simulink model "EPT"  (R2019b)
settings: Solver=FixedStepDiscrete  StartTime=0.0  StopTime=5  FixedStep=0.005  RelTol=1e-3  EnableMultiTasking=on
PreLoadFcn:
  | try, model_open; catch, disp('Error occurred while executing model pre-load callback: model_open.m'); disp('Please assure that the MATLAB working directory is set to the model directory before opening.'); end
InitFcn:
  | try, model_open; catch, end
undefined symbols (not defined in the file or in its folder): Bridge, GCM, H, ln, raptor_get_param_eval, raptor_get_safe_string, raptor_xcp_function
libraries: Raptor_lib x2810, simulink x374, hdlsllib x19
(part 28 of 45)

== system EPT/Foreground_TimeBase_5ms/CAN/CAN1_exec/BCU-CMU/CMU_Task/Tx C0-C3 ==
  Trigger : TriggerPort  VariantControl=Variant  PortDimensions=1
  Constant3 : Constant  Value=4
  Constant4 : Constant  Value=hex2dec('A0')
  Constant5 : Constant  Value=hex2dec('C0')
  raptor_can_txmsg : Raptor_lib/CAN/raptor_can_txmsg  canDefinition=struct('dbcFile', 'CMU_CMD.dbc','message', 'HostReadCMD','comment', '','signals', {{'CMU_ID','Offset','Function_Index','ID','LifeCycle'}},'enabled', [ 1 1 1 1 1;],'canBus', '''CAN1''','messageID', [ 16838272;],'idMask', [ 536870911;],'payloadMask', [],'payloadValue', [],'period', [ 0;],'mailbox', '','queueSize', [ 1;],'label', [ 1;],'ver', [ 2;],'showID', [ 0;],'showRaw', [ 0;],'fill', [ 0;],'editID', [ 0;],'signalOrder', [ 2;])  canBus='CAN1'  queueSize=1  payloadMask=[]  payloadValue=[]  period=0  showID=0  label=1  idMask=hex2dec('1FFFFFFF')  fill=0  id=16838272  showRaw=0  signalOrder=2  signalInfo={{struct('Name', 'CMU_ID','Startbit', [ 0;],'SignalSize', [ 8;],'ByteOrder', 'LittleEndian','ValueType', 'UNSIGNED','Class', 'uint8','Signed', [ 0;],'Factor', [ 1;],'Offset', [ 0;],'Min', [ 0;],'Max', [ 0;],'Units', '','Comment', '','StartBit', [ 0;]),struct('Name', 'Offset','Startbit', [ 0;],'SignalSize', [ 8;],'ByteOrder', 'LittleEndian','ValueType', 'UNSIGNED','Class', 'uint8','Signed', [ 0;],'Factor', [ 1;],'Offset', [ 0;],'Min', [ 0;],'Max', [ 0;],'Units', '','Comment', '','StartBit', [ 32;]),struct('Name', 'Function_Index','Startbit', [ 0;],'SignalSize', [ 8;],'ByteOrder', 'LittleEndian','ValueType', 'UNSIGNED','Class', 'uint8','Signed', [ 0;],'Factor', [ 1;],'Offset', [ 0;],'Min', [ 0;],'Max', [ 0;],'Units', '','Comment', '','StartBit', [ 40;]),struct('Name', 'LifeCycle','Startbit', [ 0;],'SignalSize', [ 4;],'ByteOrder', 'LittleEndian','ValueType', 'UNSIGNED','Class', 'uint8','Signed', [ 0;],'Factor', [ 1;],'Offset', [ 0;],'Min', [ 0;],'Max', [ 0;],'Units', '','Comment', '','StartBit', [ 60;]),struct('Name', 'ID','Startbit', [ 0;],'SignalSize', [ 4;],'ByteOrder', 'LittleEndian','ValueType', 'UNSIGNED','Class', 'uint8','Signed', [ 0;],'Factor', [ 1;],'Offset', [ 0;],'Min', [ 0;],'Max', [ 0;],'Units', '','Comment', '','StartBit', [ 56;])}}
      settings: SourceProductName=Raptor
  raptor_data_read2 : Raptor_lib/Data Storage/raptor_data_read  dataName='EPT_RDCMD_RC'  dataShape=Scalar  idxSource=Input  idxRow=1  idxCol=1
      settings: SourceProductName=Raptor
  raptor_data_read4 : Raptor_lib/Data Storage/raptor_data_read  dataName='EPT_RDCMD_HOST_ID'  dataShape=Scalar  idxSource=Input  idxRow=1  idxCol=1
      settings: SourceProductName=Raptor
  wires:
  raptor_data_read4/1 -> raptor_can_txmsg/4  "ID"
  Constant5/1 -> raptor_can_txmsg/3  "Function_Index"
  raptor_data_read2/1 -> raptor_can_txmsg/5  "LifeCycle"
  Constant4/1 -> raptor_can_txmsg/1  "CMU_ID"
  Constant3/1 -> raptor_can_txmsg/2  "Offset"

== system EPT/Foreground_TimeBase_5ms/CAN/CAN1_exec/BCU-CMU/CMU_Task/Tx C4-C7 ==
  Trigger : TriggerPort  VariantControl=Variant  PortDimensions=1
  Constant3 : Constant  Value=4
  Constant4 : Constant  Value=hex2dec('A0')
  Constant5 : Constant  Value=hex2dec('C4')
  raptor_can_txmsg : Raptor_lib/CAN/raptor_can_txmsg  canDefinition=struct('dbcFile', 'CMU_CMD.dbc','message', 'HostReadCMD','comment', '','signals', {{'CMU_ID','Offset','Function_Index','ID','LifeCycle'}},'enabled', [ 1 1 1 1 1;],'canBus', '''CAN1''','messageID', [ 16838272;],'idMask', [ 536870911;],'payloadMask', [],'payloadValue', [],'period', [ 0;],'mailbox', '','queueSize', [ 1;],'label', [ 1;],'ver', [ 2;],'showID', [ 0;],'showRaw', [ 0;],'fill', [ 0;],'editID', [ 0;],'signalOrder', [ 2;])  canBus='CAN1'  queueSize=1  payloadMask=[]  payloadValue=[]  period=0  showID=0  label=1  idMask=hex2dec('1FFFFFFF')  fill=0  id=16838272  showRaw=0  signalOrder=2  signalInfo={{struct('Name', 'CMU_ID','Startbit', [ 0;],'SignalSize', [ 8;],'ByteOrder', 'LittleEndian','ValueType', 'UNSIGNED','Class', 'uint8','Signed', [ 0;],'Factor', [ 1;],'Offset', [ 0;],'Min', [ 0;],'Max', [ 0;],'Units', '','Comment', '','StartBit', [ 0;]),struct('Name', 'Offset','Startbit', [ 0;],'SignalSize', [ 8;],'ByteOrder', 'LittleEndian','ValueType', 'UNSIGNED','Class', 'uint8','Signed', [ 0;],'Factor', [ 1;],'Offset', [ 0;],'Min', [ 0;],'Max', [ 0;],'Units', '','Comment', '','StartBit', [ 32;]),struct('Name', 'Function_Index','Startbit', [ 0;],'SignalSize', [ 8;],'ByteOrder', 'LittleEndian','ValueType', 'UNSIGNED','Class', 'uint8','Signed', [ 0;],'Factor', [ 1;],'Offset', [ 0;],'Min', [ 0;],'Max', [ 0;],'Units', '','Comment', '','StartBit', [ 40;]),struct('Name', 'LifeCycle','Startbit', [ 0;],'SignalSize', [ 4;],'ByteOrder', 'LittleEndian','ValueType', 'UNSIGNED','Class', 'uint8','Signed', [ 0;],'Factor', [ 1;],'Offset', [ 0;],'Min', [ 0;],'Max', [ 0;],'Units', '','Comment', '','StartBit', [ 60;]),struct('Name', 'ID','Startbit', [ 0;],'SignalSize', [ 4;],'ByteOrder', 'LittleEndian','ValueType', 'UNSIGNED','Class', 'uint8','Signed', [ 0;],'Factor', [ 1;],'Offset', [ 0;],'Min', [ 0;],'Max', [ 0;],'Units', '','Comment', '','StartBit', [ 56;])}}
      settings: SourceProductName=Raptor
  raptor_data_read2 : Raptor_lib/Data Storage/raptor_data_read  dataName='EPT_RDCMD_RC'  dataShape=Scalar  idxSource=Input  idxRow=1  idxCol=1
      settings: SourceProductName=Raptor
  raptor_data_read4 : Raptor_lib/Data Storage/raptor_data_read  dataName='EPT_RDCMD_HOST_ID'  dataShape=Scalar  idxSource=Input  idxRow=1  idxCol=1
      settings: SourceProductName=Raptor
  wires:
  raptor_data_read4/1 -> raptor_can_txmsg/4  "ID"
  Constant5/1 -> raptor_can_txmsg/3  "Function_Index"
  raptor_data_read2/1 -> raptor_can_txmsg/5  "LifeCycle"
  Constant4/1 -> raptor_can_txmsg/1  "CMU_ID"
  Constant3/1 -> raptor_can_txmsg/2  "Offset"

== system EPT/Foreground_TimeBase_5ms/CAN/CAN1_exec/IVT/CountTrigger/CycleTrigger ==
  In1 : Inport
  In2 : Inport  Port=2
  Add : Sum
  Add1 : Sum
  Add2 : Sum  Inputs=+-
  Constant1 : Constant
  Constant2 : Constant  Value=0
  Constant3 : Constant
  Data Type Conversion1 : DataTypeConversion
  Data Type Conversion2 : DataTypeConversion
  Display : Display
  Relational Operator1 : RelationalOperator  OutDataTypeStr=boolean  RndMeth=Simplest
  Scope : Scope
  Scope1 : Scope
  Scope2 : Scope
  Switch : Switch  Threshold=1
  Unit Delay : UnitDelay  SampleTime=-1  HasFrameUpgradeWarning=on
  Unit Delay1 : UnitDelay  SampleTime=-1  HasFrameUpgradeWarning=on
  Trigger : Outport  VectorParamsAs1DForOutWhenUnconnected=off
  wires:
  Constant3/1 -> Add2/2
  In2/1 -> Add2/1
  Add2/1 -> Data Type Conversion1/1
  Data Type Conversion2/1 -> Switch/2, Add/2
  Constant2/1 -> Switch/3
  Data Type Conversion1/1 -> Relational Operator1/2
  Relational Operator1/1 -> Trigger/1, Scope2/1
  Constant1/1 -> Add1/2
  Unit Delay1/1 -> Add1/1
  Add1/1 -> Display/1, Unit Delay1/1, Scope/1
  Switch/1 -> Unit Delay/1, Scope1/1, Relational Operator1/1
  Unit Delay/1 -> Add/1
  In1/1 -> Data Type Conversion2/1
  Add/1 -> Switch/1

== system EPT/Foreground_TimeBase_5ms/CAN/CAN1_exec/IVT/CountTrigger1/CycleTrigger ==
  In1 : Inport
  In2 : Inport  Port=2
  Add : Sum
  Add1 : Sum
  Add2 : Sum  Inputs=+-
  Constant1 : Constant
  Constant2 : Constant  Value=0
  Constant3 : Constant
  Data Type Conversion1 : DataTypeConversion
  Data Type Conversion2 : DataTypeConversion
  Display : Display
  Relational Operator1 : RelationalOperator  OutDataTypeStr=boolean  RndMeth=Simplest
  Scope : Scope
  Scope1 : Scope
  Scope2 : Scope
  Switch : Switch  Threshold=1
  Unit Delay : UnitDelay  SampleTime=-1  HasFrameUpgradeWarning=on
  Unit Delay1 : UnitDelay  SampleTime=-1  HasFrameUpgradeWarning=on
  Trigger : Outport  VectorParamsAs1DForOutWhenUnconnected=off
  wires:
  Add/1 -> Switch/1
  In1/1 -> Data Type Conversion2/1
  Unit Delay/1 -> Add/1
  Switch/1 -> Relational Operator1/1, Scope1/1, Unit Delay/1
  Add1/1 -> Scope/1, Unit Delay1/1, Display/1
  Unit Delay1/1 -> Add1/1
  Constant1/1 -> Add1/2
  Relational Operator1/1 -> Scope2/1, Trigger/1
  Data Type Conversion1/1 -> Relational Operator1/2
  Constant2/1 -> Switch/3
  Data Type Conversion2/1 -> Add/2, Switch/2
  Add2/1 -> Data Type Conversion1/1
  In2/1 -> Add2/1
  Constant3/1 -> Add2/2

== system EPT/Foreground_TimeBase_5ms/CAN/CAN2_exec/BCU vs ITRI//ARTC/BP-OBU Enable CTL & OP Status /BP-OBU Enable CTL ==
  Gain1 : Gain  Gain=128
  Logical Operator1 : Logic  Operator=OR  AllPortsSameDT=off  OutDataTypeStr=boolean
  Plus2 : Sum
  raptor_data_read5 : Raptor_lib/Data Storage/raptor_data_read  dataName='Flag_HV_Drive_Relay_On'  dataShape=Scalar  idxSource=Input  idxRow=1  idxCol=1
      settings: SourceProductName=Raptor
  raptor_data_read6 : Raptor_lib/Data Storage/raptor_data_read  dataName='HV_Off'  dataShape=Scalar  idxSource=Input  idxRow=1  idxCol=1
      settings: SourceProductName=Raptor
  raptor_data_read7 : Raptor_lib/Data Storage/raptor_data_read  dataName='EPT_EW_STA'  dataShape=Scalar  idxSource=Input  idxRow=1  idxCol=1
      settings: SourceProductName=Raptor
  BP-OBU Enable CTL : Outport  VectorParamsAs1DForOutWhenUnconnected=off
  wires:
  raptor_data_read6/1 -> Logical Operator1/2
  Plus2/1 -> BP-OBU Enable CTL/1
  Gain1/1 -> Plus2/2
  raptor_data_read7/1 -> Logical Operator1/1
  Logical Operator1/1 -> Gain1/1
  raptor_data_read5/1 -> Plus2/1

== system EPT/Foreground_TimeBase_5ms/CAN/CAN2_exec/BCU vs ITRI//ARTC/BP-OBU Enable CTL & OP Status /BP-OBU Output Mode ==
  Gain2 : Gain  Gain=2
  Plus1 : Sum
  raptor_data_read3 : Raptor_lib/Data Storage/raptor_data_read  dataName='Flag_Drive_Mode'  dataShape=Scalar  idxSource=Input  idxRow=1  idxCol=1
      settings: SourceProductName=Raptor
  raptor_data_read4 : Raptor_lib/Data Storage/raptor_data_read  dataName='Flag_CHG_Mode'  dataShape=Scalar  idxSource=Input  idxRow=1  idxCol=1
      settings: SourceProductName=Raptor
  BP-OBU Output Mode : Outport  VectorParamsAs1DForOutWhenUnconnected=off
  wires:
  raptor_data_read3/1 -> Plus1/1
  raptor_data_read4/1 -> Gain2/1
  Gain2/1 -> Plus1/2
  Plus1/1 -> BP-OBU Output Mode/1

== system EPT/Foreground_TimeBase_5ms/CAN/CAN2_exec/BCU vs ITRI//ARTC/BP-OBU Enable CTL & OP Status /BP-OBU_Enable Mode ==
  note: Notes : Mode EN
      | - Not Ready==00b
      | - Drive EN ==01b
      | - CHG EN ==10b
      | - Ready ==11b
  Gain1 : Gain  Gain=64
  Gain3 : Gain  Gain=16
  Gain6 : Gain  Gain=32
  Plus2 : Sum  Inputs=++++
  raptor_data_read1 : Raptor_lib/Data Storage/raptor_data_read  dataName='HV_Off'  dataShape=Scalar  idxSource=Input  idxRow=1  idxCol=1
      settings: SourceProductName=Raptor
  raptor_data_read2 : Raptor_lib/Data Storage/raptor_data_read  dataName='Warning_EndOfDischarge'  dataShape=Scalar  idxSource=Input  idxRow=1  idxCol=1
      settings: SourceProductName=Raptor
  raptor_data_read3 : Raptor_lib/Data Storage/raptor_data_read  dataName='Warning_EndOfCharge'  dataShape=Scalar  idxSource=Input  idxRow=1  idxCol=1
      settings: SourceProductName=Raptor
  raptor_data_read6 : Raptor_lib/Data Storage/raptor_data_read  dataName='EPT_VEH_MODE_STA'  dataShape=Scalar  idxSource=Input  idxRow=1  idxCol=1
      settings: SourceProductName=Raptor
  BP-OBU_Enable Mode : Outport  VectorParamsAs1DForOutWhenUnconnected=off
  wires:
  Gain3/1 -> Plus2/2
  raptor_data_read3/1 -> Gain6/1
  raptor_data_read6/1 -> Plus2/1
  Gain6/1 -> Plus2/3
  raptor_data_read2/1 -> Gain3/1
  Plus2/1 -> BP-OBU_Enable Mode/1
  raptor_data_read1/1 -> Gain1/1
  Gain1/1 -> Plus2/4

== system EPT/Foreground_TimeBase_5ms/CAN/CAN2_exec/BCU vs ITRI//ARTC/BP-OBU Enable CTL & OP Status /BP-OBU_HV CTL Mode ==
  Gain1 : Gain  Gain=2
  Gain2 : Gain  Gain=128
  Gain3 : Gain  Gain=4
  Gain4 : Gain  Gain=16
  Gain5 : Gain  Gain=32
  Gain6 : Gain  Gain=8
  Logical Operator : Logic  AllPortsSameDT=off  OutDataTypeStr=boolean
  Logical Operator1 : Logic  AllPortsSameDT=off  OutDataTypeStr=boolean
  Plus2 : Sum  Inputs=+++++++
  raptor_data_read1 : Raptor_lib/Data Storage/raptor_data_read  dataName='Fault_HV_Setup_Fault'  dataShape=Scalar  idxSource=Input  idxRow=1  idxCol=1
      settings: SourceProductName=Raptor
  raptor_data_read10 : Raptor_lib/Data Storage/raptor_data_read  dataName='Relay_CHG_OBC'  dataShape=Scalar  idxSource=Input  idxRow=1  idxCol=1
      settings: SourceProductName=Raptor
  raptor_data_read5 : Raptor_lib/Data Storage/raptor_data_read  dataName='Flag_HV_Drive_Relay_On'  dataShape=Scalar  idxSource=Input  idxRow=1  idxCol=1
      settings: SourceProductName=Raptor
  raptor_data_read6 : Raptor_lib/Data Storage/raptor_data_read  dataName='Flag_PreCharge_Relay_On'  dataShape=Scalar  idxSource=Input  idxRow=1  idxCol=1
      settings: SourceProductName=Raptor
  raptor_data_read7 : Raptor_lib/Data Storage/raptor_data_read  dataName='Flag_Charger_Relay_On'  dataShape=Scalar  idxSource=Input  idxRow=1  idxCol=1
      settings: SourceProductName=Raptor
  raptor_data_read8 : Raptor_lib/Data Storage/raptor_data_read  dataName='Flag_HV_Negative_Relay_On'  dataShape=Scalar  idxSource=Input  idxRow=1  idxCol=1
      settings: SourceProductName=Raptor
  raptor_data_read9 : Raptor_lib/Data Storage/raptor_data_read  dataName='Relay_MCU'  dataShape=Scalar  idxSource=Input  idxRow=1  idxCol=1
      settings: SourceProductName=Raptor
  BP-OBU_HV CTL Mode : Outport  VectorParamsAs1DForOutWhenUnconnected=off
  wires:
  Plus2/1 -> BP-OBU_HV CTL Mode/1
  raptor_data_read8/1 -> Gain3/1
  Logical Operator1/1 -> Gain6/1
  Logical Operator/1 -> Gain5/1
  Gain4/1 -> Plus2/5
  raptor_data_read9/1 -> Logical Operator1/2
  raptor_data_read10/1 -> Logical Operator/2
  raptor_data_read7/1 -> Gain4/1
  raptor_data_read5/1 -> Logical Operator1/1, Logical Operator/1, Gain1/1
  Gain6/1 -> Plus2/4
  Gain3/1 -> Plus2/3
  raptor_data_read6/1 -> Plus2/1
  Gain5/1 -> Plus2/6
  Gain1/1 -> Plus2/2
  raptor_data_read1/1 -> Gain2/1
  Gain2/1 -> Plus2/7

== system EPT/Foreground_TimeBase_5ms/CAN/CAN2_exec/BCU vs ITRI//ARTC/BP-OBU Enable CTL & OP Status /BP-OBU_OP Mode ==
  Constant1 : Constant  Value=0
  Gain1 : Gain  Gain=2
  Gain2 : Gain  Gain=64
  Gain3 : Gain  Gain=4
  Gain4 : Gain  Gain=16
  Gain5 : Gain  Gain=32
  Gain6 : Gain  Gain=8
  Gain7 : Gain  Gain=128
  Logical Operator1 : Logic  Operator=NOR  AllPortsSameDT=off  OutDataTypeStr=boolean
  Logical Operator2 : Logic  AllPortsSameDT=off  OutDataTypeStr=boolean
  NOT : Logic  Operator=NOT  IconShape=distinctive  AllPortsSameDT=off  OutDataTypeStr=boolean
  NOT1 : Logic  Operator=NOT  IconShape=distinctive  AllPortsSameDT=off  OutDataTypeStr=boolean
  Plus2 : Sum  Inputs=++++++++
  raptor_data_read1 : Raptor_lib/Data Storage/raptor_data_read  dataName='Flag_PreCharge_Relay_On'  dataShape=Scalar  idxSource=Input  idxRow=1  idxCol=1
      settings: SourceProductName=Raptor
  raptor_data_read12 : Raptor_lib/Data Storage/raptor_data_read  dataName='HV_Off'  dataShape=Scalar  idxSource=Input  idxRow=1  idxCol=1
      settings: SourceProductName=Raptor
  raptor_data_read2 : Raptor_lib/Data Storage/raptor_data_read  dataName='Flag_HV_Negative_Relay_On'  dataShape=Scalar  idxSource=Input  idxRow=1  idxCol=1
      settings: SourceProductName=Raptor
  raptor_data_read3 : Raptor_lib/Data Storage/raptor_data_read  dataName='Flag_HV_Drive_Relay_On'  dataShape=Scalar  idxSource=Input  idxRow=1  idxCol=1
      settings: SourceProductName=Raptor
  raptor_data_read4 : Raptor_lib/Data Storage/raptor_data_read  dataName='EPT_EW_STA'  dataShape=Scalar  idxSource=Input  idxRow=1  idxCol=1
      settings: SourceProductName=Raptor
  raptor_data_read6 : Raptor_lib/Data Storage/raptor_data_read  dataName='HV_Off'  dataShape=Scalar  idxSource=Input  idxRow=1  idxCol=1
      settings: SourceProductName=Raptor
  raptor_data_read7 : Raptor_lib/Data Storage/raptor_data_read  dataName='EPT_EW_STA'  dataShape=Scalar  idxSource=Input  idxRow=1  idxCol=1
      settings: SourceProductName=Raptor
  BP-OBU_OP Mode : Outport  VectorParamsAs1DForOutWhenUnconnected=off
  wires:
  Gain7/1 -> Plus2/8
  Gain2/1 -> Plus2/7
  raptor_data_read12/1 -> Gain4/1
  raptor_data_read3/1 -> Gain6/1
  Logical Operator2/1 -> Gain1/1
  NOT/1 -> Logical Operator2/2
  raptor_data_read2/1 -> NOT/1
  raptor_data_read1/1 -> Gain3/1
  raptor_data_read7/1 -> Logical Operator1/1
  Logical Operator1/1 -> Logical Operator2/1
  raptor_data_read6/1 -> Logical Operator1/2
  Plus2/1 -> BP-OBU_OP Mode/1
  Gain4/1 -> Plus2/5
  Gain6/1 -> Plus2/4
  Gain3/1 -> Plus2/3
  Constant1/1 -> Gain7/1, Gain2/1, Gain5/1
  Gain5/1 -> Plus2/6
  Gain1/1 -> Plus2/2
  NOT1/1 -> Plus2/1
  raptor_data_read4/1 -> NOT1/1

== system EPT/Foreground_TimeBase_5ms/CAN/CAN2_exec/BCU vs ITRI//ARTC/BP-OBU Enable CTL & OP Status /EPT Status Bitmap ==
  Gain : Gain  Gain=128
  Plus : Sum
  raptor_data_read1 : Raptor_lib/Data Storage/raptor_data_read  dataName='EPT_READY'  dataShape=Scalar  idxSource=Input  idxRow=1  idxCol=1
      settings: SourceProductName=Raptor
  raptor_data_read2 : Raptor_lib/Data Storage/raptor_data_read  dataName='EPT_EW_STA'  dataShape=Scalar  idxSource=Input  idxRow=1  idxCol=1
      settings: SourceProductName=Raptor
  EPT Status Bitmap : Outport  VectorParamsAs1DForOutWhenUnconnected=off
  wires:
  raptor_data_read1/1 -> Plus/1
  Plus/1 -> EPT Status Bitmap/1
  raptor_data_read2/1 -> Gain/1
  Gain/1 -> Plus/2

== system EPT/Foreground_TimeBase_5ms/CAN/CAN2_exec/BCU vs ITRI//ARTC/CountTrigger1/CycleTrigger ==
  In1 : Inport
  In2 : Inport  Port=2
  Add : Sum
  Add1 : Sum
  Add2 : Sum  Inputs=+-
  Constant1 : Constant
  Constant2 : Constant  Value=0
  Constant3 : Constant
  Data Type Conversion1 : DataTypeConversion
  Data Type Conversion2 : DataTypeConversion
  Display : Display
  Relational Operator1 : RelationalOperator  OutDataTypeStr=boolean  RndMeth=Simplest
  Scope : Scope
  Scope1 : Scope
  Scope2 : Scope
  Switch : Switch  Threshold=1
  Unit Delay : UnitDelay  SampleTime=-1  HasFrameUpgradeWarning=on
  Unit Delay1 : UnitDelay  SampleTime=-1  HasFrameUpgradeWarning=on
  Trigger : Outport  VectorParamsAs1DForOutWhenUnconnected=off
  wires:
  Add/1 -> Switch/1
  In1/1 -> Data Type Conversion2/1
  Unit Delay/1 -> Add/1
  Switch/1 -> Relational Operator1/1, Scope1/1, Unit Delay/1
  Add1/1 -> Scope/1, Unit Delay1/1, Display/1
  Unit Delay1/1 -> Add1/1
  Constant1/1 -> Add1/2
  Relational Operator1/1 -> Scope2/1, Trigger/1
  Data Type Conversion1/1 -> Relational Operator1/2
  Constant2/1 -> Switch/3
  Data Type Conversion2/1 -> Add/2, Switch/2
  Add2/1 -> Data Type Conversion1/1
  In2/1 -> Add2/1
  Constant3/1 -> Add2/2

== system EPT/Foreground_TimeBase_5ms/CAN/CAN2_exec/ECHS/CountTrigger/CycleTrigger ==
  In1 : Inport
  In2 : Inport  Port=2
  Add : Sum
  Add1 : Sum
  Add2 : Sum  Inputs=+-
  Constant1 : Constant
  Constant2 : Constant  Value=0
  Constant3 : Constant
  Data Type Conversion1 : DataTypeConversion
  Data Type Conversion2 : DataTypeConversion
  Display : Display
  Relational Operator1 : RelationalOperator  OutDataTypeStr=boolean  RndMeth=Simplest
  Scope : Scope
  Scope1 : Scope
  Scope2 : Scope
  Switch : Switch  Threshold=1
  Unit Delay : UnitDelay  SampleTime=-1  HasFrameUpgradeWarning=on
  Unit Delay1 : UnitDelay  SampleTime=-1  HasFrameUpgradeWarning=on
  Trigger : Outport  VectorParamsAs1DForOutWhenUnconnected=off
  wires:
  Add/1 -> Switch/1
  In1/1 -> Data Type Conversion2/1
  Unit Delay/1 -> Add/1
  Switch/1 -> Relational Operator1/1, Scope1/1, Unit Delay/1
  Add1/1 -> Scope/1, Unit Delay1/1, Display/1
  Unit Delay1/1 -> Add1/1
  Constant1/1 -> Add1/2
  Relational Operator1/1 -> Scope2/1, Trigger/1
  Data Type Conversion1/1 -> Relational Operator1/2
  Constant2/1 -> Switch/3
  Data Type Conversion2/1 -> Add/2, Switch/2
  Add2/1 -> Data Type Conversion1/1
  In2/1 -> Add2/1
  Constant3/1 -> Add2/2

== system EPT/Foreground_TimeBase_5ms/CAN/CAN2_exec/ECHS/EPT2ECHS_RX/10ms_exec ==
  0xC10F4D0_DBC : Subsystem

== system EPT/Foreground_TimeBase_5ms/CAN/CAN2_exec/ECHS/EPT2ECHS_TX/100ms_exec ==
  0x1851FFF4_DBC : Subsystem
  0x1852FFF4_DBC : Subsystem
  0x1853FFF4_DBC : Subsystem
  Constant12 : Constant  Value=10
  CountTrigger : Subsystem
  Delay : Delay
  Delay1 : Delay
  wires:
  Constant12/1 -> CountTrigger/1(Counter)
  CountTrigger/1(Tirgger) -> 0x1853FFF4_DBC/Trigger, Delay1/1
  Delay/1 -> 0x1851FFF4_DBC/Trigger
  Delay1/1 -> Delay/1, 0x1852FFF4_DBC/Trigger

== system EPT/Foreground_TimeBase_5ms/CAN/CAN2_exec/ECHS/EPT2ECHS_TX/10ms_exec ==
  0xC10D0F4_DBC : Subsystem

== system EPT/Foreground_TimeBase_5ms/CAN/CAN2_exec/ECHS/EPT2ECHS_TX/500ms_exec ==
  0x1820FFF4_DBC : Subsystem
  Constant12 : Constant  Value=50
  CountTrigger : Subsystem
  wires:
  CountTrigger/1(Tirgger) -> 0x1820FFF4_DBC/Trigger
  Constant12/1 -> CountTrigger/1(Counter)

== system EPT/Foreground_TimeBase_5ms/CAN/CAN2_exec/IVT2/Coulomb Counting Method1/20ms ==
  Ampere input : Inport
  RC input : Inport  Port=2
  Trigger : TriggerPort  VariantControl=Variant  PortDimensions=1
  Add2 : Sum
  Add3 : Sum
  Constant1 : Constant  Value=0
  Constant3 : Constant  Value=50
  Constant4 : Constant  Value=3600
  CountTrigger3 : Subsystem
  Delay1 : Delay  DelayLength=1  InitialCondition=0
  Divide1 : Product  Inputs=*/
  Divide3 : Product  Inputs=*/
  Switch1 : Switch  Criteria=u2 > Threshold
  Switch2 : Switch  Criteria=u2 > Threshold
  RC : Outport
  wires:
  Ampere input/1 -> Divide3/1
  Divide3/1 -> Add2/1
  Switch2/1 -> Divide1/1
  Delay1/1 -> Add2/2
  Switch1/1 -> Delay1/1
  Add2/1 -> Switch1/3, Switch2/1
  CountTrigger3/1(Tirgger) -> Switch2/2, Switch1/2
  Constant4/1 -> Divide1/2
  Constant1/1 -> Switch1/1, Switch2/3
  Divide1/1 -> Add3/1
  RC input/1 -> Add3/2
  Constant3/1 -> Divide3/2, CountTrigger3/1(Counter)
  Add3/1 -> RC/1

== system EPT/Foreground_TimeBase_5ms/CAN/CAN2_exec/IVT2/Coulomb Counting Method1/CountTrigger ==
  Counter : Inport
  Constant1 : Constant  Value=0
  Constant3 : Constant
  CycleTrigger : Subsystem
  Switch : Switch  Threshold=1
  Unit Delay1 : UnitDelay  SampleTime=-1  HasFrameUpgradeWarning=on
  Unit Delay2 : UnitDelay  SampleTime=-1  HasFrameUpgradeWarning=on
  Tirgger : Outport  VectorParamsAs1DForOutWhenUnconnected=off
  wires:
  Unit Delay2/1 -> Tirgger/1
  Unit Delay1/1 -> CycleTrigger/1(In1)
  CycleTrigger/1(Trigger) -> Unit Delay2/1, Switch/2
  Counter/1 -> CycleTrigger/2(In2)
  Constant1/1 -> Switch/1
  Constant3/1 -> Switch/3
  Switch/1 -> Unit Delay1/1

== system EPT/Foreground_TimeBase_5ms/CAN/CAN2_exec/IVT2/CountTrigger/CycleTrigger ==
  In1 : Inport
  In2 : Inport  Port=2
  Add : Sum
  Add1 : Sum
  Add2 : Sum  Inputs=+-
  Constant1 : Constant
  Constant2 : Constant  Value=0
  Constant3 : Constant
  Data Type Conversion1 : DataTypeConversion
  Data Type Conversion2 : DataTypeConversion
  Display : Display
  Relational Operator1 : RelationalOperator  OutDataTypeStr=boolean  RndMeth=Simplest
  Scope : Scope
  Scope1 : Scope
  Scope2 : Scope
  Switch : Switch  Threshold=1
  Unit Delay : UnitDelay  SampleTime=-1  HasFrameUpgradeWarning=on
  Unit Delay1 : UnitDelay  SampleTime=-1  HasFrameUpgradeWarning=on
  Trigger : Outport  VectorParamsAs1DForOutWhenUnconnected=off
  wires:
  Constant3/1 -> Add2/2
  In2/1 -> Add2/1
  Add2/1 -> Data Type Conversion1/1
  Data Type Conversion2/1 -> Switch/2, Add/2
  Constant2/1 -> Switch/3
  Data Type Conversion1/1 -> Relational Operator1/2
  Relational Operator1/1 -> Trigger/1, Scope2/1
  Constant1/1 -> Add1/2
  Unit Delay1/1 -> Add1/1
  Add1/1 -> Display/1, Unit Delay1/1, Scope/1
  Switch/1 -> Unit Delay/1, Scope1/1, Relational Operator1/1
  Unit Delay/1 -> Add/1
  In1/1 -> Data Type Conversion2/1
  Add/1 -> Switch/1

== system EPT/Foreground_TimeBase_5ms/CAN/CAN2_exec/IVT2/CountTrigger1/CycleTrigger ==
  In1 : Inport
  In2 : Inport  Port=2
  Add : Sum
  Add1 : Sum
  Add2 : Sum  Inputs=+-
  Constant1 : Constant
  Constant2 : Constant  Value=0
  Constant3 : Constant
  Data Type Conversion1 : DataTypeConversion
  Data Type Conversion2 : DataTypeConversion
  Display : Display
  Relational Operator1 : RelationalOperator  OutDataTypeStr=boolean  RndMeth=Simplest
  Scope : Scope
  Scope1 : Scope
  Scope2 : Scope
  Switch : Switch  Threshold=1
  Unit Delay : UnitDelay  SampleTime=-1  HasFrameUpgradeWarning=on
  Unit Delay1 : UnitDelay  SampleTime=-1  HasFrameUpgradeWarning=on
  Trigger : Outport  VectorParamsAs1DForOutWhenUnconnected=off
  wires:
  Add/1 -> Switch/1
  In1/1 -> Data Type Conversion2/1
  Unit Delay/1 -> Add/1
  Switch/1 -> Relational Operator1/1, Scope1/1, Unit Delay/1
  Add1/1 -> Scope/1, Unit Delay1/1, Display/1
  Unit Delay1/1 -> Add1/1
  Constant1/1 -> Add1/2
  Relational Operator1/1 -> Scope2/1, Trigger/1
  Data Type Conversion1/1 -> Relational Operator1/2
  Constant2/1 -> Switch/3
  Data Type Conversion2/1 -> Add/2, Switch/2
  Add2/1 -> Data Type Conversion1/1
  In2/1 -> Add2/1
  Constant3/1 -> Add2/2

== system EPT/Foreground_TimeBase_5ms/CAN/CAN2_exec/IVT2/Delay2/CycleTrigger ==
  In1 : Inport
  In2 : Inport  Port=2
  Add : Sum
  Add2 : Sum  Inputs=+-
  Constant2 : Constant  Value=0
  Constant3 : Constant
  Data Type Conversion1 : DataTypeConversion
  Data Type Conversion2 : DataTypeConversion
  Relational Operator1 : RelationalOperator  OutDataTypeStr=boolean  RndMeth=Simplest
  Saturation : Saturate  UpperLimit=inf  LowerLimit=2
  Switch : Switch  Threshold=1
  Unit Delay : UnitDelay  SampleTime=-1  HasFrameUpgradeWarning=on
  Trigger : Outport  VectorParamsAs1DForOutWhenUnconnected=off
  wires:
  Saturation/1 -> Add2/1
  Add/1 -> Switch/1
  In1/1 -> Data Type Conversion2/1
  Unit Delay/1 -> Add/1
  Switch/1 -> Relational Operator1/1, Unit Delay/1
  Relational Operator1/1 -> Trigger/1
  Data Type Conversion1/1 -> Relational Operator1/2
  Constant2/1 -> Switch/3
  Data Type Conversion2/1 -> Add/2, Switch/2
  Add2/1 -> Data Type Conversion1/1
  In2/1 -> Saturation/1
  Constant3/1 -> Add2/2

== system EPT/Foreground_TimeBase_5ms/CAN/CAN2_exec/IVT2/Delay3/CycleTrigger ==
  In1 : Inport
  In2 : Inport  Port=2
  Add : Sum
  Add2 : Sum  Inputs=+-
  Constant2 : Constant  Value=0
  Constant3 : Constant
  Data Type Conversion1 : DataTypeConversion
  Data Type Conversion2 : DataTypeConversion
  Relational Operator1 : RelationalOperator  OutDataTypeStr=boolean  RndMeth=Simplest
  Saturation : Saturate  UpperLimit=inf  LowerLimit=2
  Switch : Switch  Threshold=1
  Unit Delay : UnitDelay  SampleTime=-1  HasFrameUpgradeWarning=on
  Trigger : Outport  VectorParamsAs1DForOutWhenUnconnected=off
  wires:
  Constant3/1 -> Add2/2
  In2/1 -> Saturation/1
  Add2/1 -> Data Type Conversion1/1
  Data Type Conversion2/1 -> Switch/2, Add/2
  Constant2/1 -> Switch/3
  Data Type Conversion1/1 -> Relational Operator1/2
  Relational Operator1/1 -> Trigger/1
  Switch/1 -> Unit Delay/1, Relational Operator1/1
  Unit Delay/1 -> Add/1
  In1/1 -> Data Type Conversion2/1
  Add/1 -> Switch/1
  Saturation/1 -> Add2/1

== system EPT/Foreground_TimeBase_5ms/CAN/CAN2_exec/Remote DA /CountTrigger/CycleTrigger ==
  In1 : Inport
  In2 : Inport  Port=2
  Add : Sum
  Add1 : Sum
  Add2 : Sum  Inputs=+-
  Constant1 : Constant
  Constant2 : Constant  Value=0
  Constant3 : Constant
  Data Type Conversion1 : DataTypeConversion
  Data Type Conversion2 : DataTypeConversion
  Display : Display
  Relational Operator1 : RelationalOperator  OutDataTypeStr=boolean  RndMeth=Simplest
  Scope : Scope
  Scope1 : Scope
  Scope2 : Scope
  Switch : Switch  Threshold=1
  Unit Delay : UnitDelay  SampleTime=-1  HasFrameUpgradeWarning=on
  Unit Delay1 : UnitDelay  SampleTime=-1  HasFrameUpgradeWarning=on
  Trigger : Outport  VectorParamsAs1DForOutWhenUnconnected=off
  wires:
  Constant3/1 -> Add2/2
  In2/1 -> Add2/1
  Add2/1 -> Data Type Conversion1/1
  Data Type Conversion2/1 -> Switch/2, Add/2
  Constant2/1 -> Switch/3
  Data Type Conversion1/1 -> Relational Operator1/2
  Relational Operator1/1 -> Trigger/1, Scope2/1
  Constant1/1 -> Add1/2
  Unit Delay1/1 -> Add1/1
  Add1/1 -> Display/1, Unit Delay1/1, Scope/1
  Switch/1 -> Unit Delay/1, Scope1/1, Relational Operator1/1
  Unit Delay/1 -> Add/1
  In1/1 -> Data Type Conversion2/1
  Add/1 -> Switch/1

== system EPT/Foreground_TimeBase_5ms/CAN/CAN2_exec/Remote DA /Remote DA Status G22 (ESS-OBU#3)/Tcell Min//Max ==
  Mux : Mux  Inputs=30
  Sort : MATLAB Function  TreatAsAtomicUnit=on
  raptor_data_read : Raptor_lib/Data Storage/raptor_data_read  dataName='CMU1_CELL01_TEMP'  dataShape=Scalar  idxSource=Input  idxRow=1  idxCol=1
      settings: SourceProductName=Raptor
  raptor_data_read1 : Raptor_lib/Data Storage/raptor_data_read  dataName='CMU1_CELL02_TEMP'  dataShape=Scalar  idxSource=Input  idxRow=1  idxCol=1
      settings: SourceProductName=Raptor
  raptor_data_read10 : Raptor_lib/Data Storage/raptor_data_read  dataName='CMU1_CELL11_TEMP'  dataShape=Scalar  idxSource=Input  idxRow=1  idxCol=1
      settings: SourceProductName=Raptor
  raptor_data_read11 : Raptor_lib/Data Storage/raptor_data_read  dataName='CMU1_CELL12_TEMP'  dataShape=Scalar  idxSource=Input  idxRow=1  idxCol=1
      settings: SourceProductName=Raptor
  raptor_data_read12 : Raptor_lib/Data Storage/raptor_data_read  dataName='CMU1_CELL13_TEMP'  dataShape=Scalar  idxSource=Input  idxRow=1  idxCol=1
      settings: SourceProductName=Raptor
  raptor_data_read13 : Raptor_lib/Data Storage/raptor_data_read  dataName='CMU1_CELL14_TEMP'  dataShape=Scalar  idxSource=Input  idxRow=1  idxCol=1
      settings: SourceProductName=Raptor
  raptor_data_read14 : Raptor_lib/Data Storage/raptor_data_read  dataName='CMU1_CELL15_TEMP'  dataShape=Scalar  idxSource=Input  idxRow=1  idxCol=1
      settings: SourceProductName=Raptor
  raptor_data_read2 : Raptor_lib/Data Storage/raptor_data_read  dataName='CMU1_CELL03_TEMP'  dataShape=Scalar  idxSource=Input  idxRow=1  idxCol=1
      settings: SourceProductName=Raptor
  raptor_data_read3 : Raptor_lib/Data Storage/raptor_data_read  dataName='CMU1_CELL04_TEMP'  dataShape=Scalar  idxSource=Input  idxRow=1  idxCol=1
      settings: SourceProductName=Raptor
  raptor_data_read30 : Raptor_lib/Data Storage/raptor_data_read  dataName='CMU2_CELL01_TEMP'  dataShape=Scalar  idxSource=Input  idxRow=1  idxCol=1
      settings: SourceProductName=Raptor
  raptor_data_read31 : Raptor_lib/Data Storage/raptor_data_read  dataName='CMU2_CELL02_TEMP'  dataShape=Scalar  idxSource=Input  idxRow=1  idxCol=1
      settings: SourceProductName=Raptor
  raptor_data_read32 : Raptor_lib/Data Storage/raptor_data_read  dataName='CMU2_CELL11_TEMP'  dataShape=Scalar  idxSource=Input  idxRow=1  idxCol=1
      settings: SourceProductName=Raptor
  raptor_data_read33 : Raptor_lib/Data Storage/raptor_data_read  dataName='CMU2_CELL12_TEMP'  dataShape=Scalar  idxSource=Input  idxRow=1  idxCol=1
      settings: SourceProductName=Raptor
  raptor_data_read34 : Raptor_lib/Data Storage/raptor_data_read  dataName='CMU2_CELL13_TEMP'  dataShape=Scalar  idxSource=Input  idxRow=1  idxCol=1
      settings: SourceProductName=Raptor
  raptor_data_read35 : Raptor_lib/Data Storage/raptor_data_read  dataName='CMU2_CELL14_TEMP'  dataShape=Scalar  idxSource=Input  idxRow=1  idxCol=1
      settings: SourceProductName=Raptor
  raptor_data_read36 : Raptor_lib/Data Storage/raptor_data_read  dataName='CMU2_CELL15_TEMP'  dataShape=Scalar  idxSource=Input  idxRow=1  idxCol=1
      settings: SourceProductName=Raptor
  raptor_data_read4 : Raptor_lib/Data Storage/raptor_data_read  dataName='CMU1_CELL05_TEMP'  dataShape=Scalar  idxSource=Input  idxRow=1  idxCol=1
      settings: SourceProductName=Raptor
  raptor_data_read42 : Raptor_lib/Data Storage/raptor_data_read  dataName='CMU2_CELL03_TEMP'  dataShape=Scalar  idxSource=Input  idxRow=1  idxCol=1
      settings: SourceProductName=Raptor
  raptor_data_read5 : Raptor_lib/Data Storage/raptor_data_read  dataName='CMU1_CELL06_TEMP'  dataShape=Scalar  idxSource=Input  idxRow=1  idxCol=1
      settings: SourceProductName=Raptor
  raptor_data_read53 : Raptor_lib/Data Storage/raptor_data_read  dataName='CMU2_CELL04_TEMP'  dataShape=Scalar  idxSource=Input  idxRow=1  idxCol=1
      settings: SourceProductName=Raptor
  raptor_data_read54 : Raptor_lib/Data Storage/raptor_data_read  dataName='CMU2_CELL05_TEMP'  dataShape=Scalar  idxSource=Input  idxRow=1  idxCol=1
      settings: SourceProductName=Raptor
  raptor_data_read55 : Raptor_lib/Data Storage/raptor_data_read  dataName='CMU2_CELL06_TEMP'  dataShape=Scalar  idxSource=Input  idxRow=1  idxCol=1
      settings: SourceProductName=Raptor
  raptor_data_read56 : Raptor_lib/Data Storage/raptor_data_read  dataName='CMU2_CELL07_TEMP'  dataShape=Scalar  idxSource=Input  idxRow=1  idxCol=1
      settings: SourceProductName=Raptor
  raptor_data_read57 : Raptor_lib/Data Storage/raptor_data_read  dataName='CMU2_CELL08_TEMP'  dataShape=Scalar  idxSource=Input  idxRow=1  idxCol=1
      settings: SourceProductName=Raptor
  raptor_data_read58 : Raptor_lib/Data Storage/raptor_data_read  dataName='CMU2_CELL09_TEMP'  dataShape=Scalar  idxSource=Input  idxRow=1  idxCol=1
      settings: SourceProductName=Raptor
  raptor_data_read59 : Raptor_lib/Data Storage/raptor_data_read  dataName='CMU2_CELL10_TEMP'  dataShape=Scalar  idxSource=Input  idxRow=1  idxCol=1
      settings: SourceProductName=Raptor
  raptor_data_read6 : Raptor_lib/Data Storage/raptor_data_read  dataName='CMU1_CELL07_TEMP'  dataShape=Scalar  idxSource=Input  idxRow=1  idxCol=1
      settings: SourceProductName=Raptor
  raptor_data_read7 : Raptor_lib/Data Storage/raptor_data_read  dataName='CMU1_CELL08_TEMP'  dataShape=Scalar  idxSource=Input  idxRow=1  idxCol=1
      settings: SourceProductName=Raptor
  raptor_data_read8 : Raptor_lib/Data Storage/raptor_data_read  dataName='CMU1_CELL09_TEMP'  dataShape=Scalar  idxSource=Input  idxRow=1  idxCol=1
      settings: SourceProductName=Raptor
  raptor_data_read9 : Raptor_lib/Data Storage/raptor_data_read  dataName='CMU1_CELL10_TEMP'  dataShape=Scalar  idxSource=Input  idxRow=1  idxCol=1
      settings: SourceProductName=Raptor
  Max : Outport
  Min : Outport  Port=2
  Max Order : Outport  Port=3
  Min Order : Outport  Port=4
  wires:
  Sort/4(Min_order) -> Min Order/1
  Sort/3(Max_order) -> Max Order/1
  raptor_data_read36/1 -> Mux/30
  raptor_data_read35/1 -> Mux/29
  raptor_data_read34/1 -> Mux/28
  raptor_data_read33/1 -> Mux/27
  raptor_data_read32/1 -> Mux/26
  raptor_data_read59/1 -> Mux/25
  raptor_data_read58/1 -> Mux/24
  raptor_data_read57/1 -> Mux/23
  raptor_data_read56/1 -> Mux/22
  raptor_data_read55/1 -> Mux/21
  raptor_data_read54/1 -> Mux/20
  raptor_data_read53/1 -> Mux/19
  raptor_data_read42/1 -> Mux/18
  raptor_data_read31/1 -> Mux/17
  raptor_data_read30/1 -> Mux/16
  raptor_data_read14/1 -> Mux/15
  raptor_data_read13/1 -> Mux/14
  raptor_data_read12/1 -> Mux/13
  raptor_data_read11/1 -> Mux/12
  raptor_data_read10/1 -> Mux/11
  raptor_data_read9/1 -> Mux/10
  raptor_data_read8/1 -> Mux/9
  raptor_data_read7/1 -> Mux/8
  raptor_data_read6/1 -> Mux/7
  raptor_data_read5/1 -> Mux/6
  raptor_data_read4/1 -> Mux/5
  raptor_data_read3/1 -> Mux/4
  raptor_data_read2/1 -> Mux/3
  raptor_data_read1/1 -> Mux/2
  raptor_data_read/1 -> Mux/1
  Sort/1(Max) -> Max/1
  Mux/1 -> Sort/1(array)
  Sort/2(Min) -> Min/1

== system EPT/Foreground_TimeBase_5ms/CAN/CAN2_exec/Remote DA /Remote DA Status G22 (ESS-OBU#3)/Vcell Min//Max ==
  Mux : Mux  Inputs=30
  Sort : MATLAB Function  TreatAsAtomicUnit=on
  raptor_data_read : Raptor_lib/Data Storage/raptor_data_read  dataName='CMU1_CELL01_VOLT'  dataShape=Scalar  idxSource=Input  idxRow=1  idxCol=1
      settings: SourceProductName=Raptor
  raptor_data_read1 : Raptor_lib/Data Storage/raptor_data_read  dataName='CMU1_CELL02_VOLT'  dataShape=Scalar  idxSource=Input  idxRow=1  idxCol=1
      settings: SourceProductName=Raptor
  raptor_data_read10 : Raptor_lib/Data Storage/raptor_data_read  dataName='CMU1_CELL11_VOLT'  dataShape=Scalar  idxSource=Input  idxRow=1  idxCol=1
      settings: SourceProductName=Raptor
  raptor_data_read11 : Raptor_lib/Data Storage/raptor_data_read  dataName='CMU1_CELL12_VOLT'  dataShape=Scalar  idxSource=Input  idxRow=1  idxCol=1
      settings: SourceProductName=Raptor
  raptor_data_read12 : Raptor_lib/Data Storage/raptor_data_read  dataName='CMU1_CELL13_VOLT'  dataShape=Scalar  idxSource=Input  idxRow=1  idxCol=1
      settings: SourceProductName=Raptor
  raptor_data_read13 : Raptor_lib/Data Storage/raptor_data_read  dataName='CMU1_CELL14_VOLT'  dataShape=Scalar  idxSource=Input  idxRow=1  idxCol=1
      settings: SourceProductName=Raptor
  raptor_data_read14 : Raptor_lib/Data Storage/raptor_data_read  dataName='CMU1_CELL15_VOLT'  dataShape=Scalar  idxSource=Input  idxRow=1  idxCol=1
      settings: SourceProductName=Raptor
  raptor_data_read2 : Raptor_lib/Data Storage/raptor_data_read  dataName='CMU1_CELL03_VOLT'  dataShape=Scalar  idxSource=Input  idxRow=1  idxCol=1
      settings: SourceProductName=Raptor
  raptor_data_read3 : Raptor_lib/Data Storage/raptor_data_read  dataName='CMU1_CELL04_VOLT'  dataShape=Scalar  idxSource=Input  idxRow=1  idxCol=1
      settings: SourceProductName=Raptor
  raptor_data_read30 : Raptor_lib/Data Storage/raptor_data_read  dataName='CMU2_CELL01_VOLT'  dataShape=Scalar  idxSource=Input  idxRow=1  idxCol=1
      settings: SourceProductName=Raptor
  raptor_data_read31 : Raptor_lib/Data Storage/raptor_data_read  dataName='CMU2_CELL02_VOLT'  dataShape=Scalar  idxSource=Input  idxRow=1  idxCol=1
      settings: SourceProductName=Raptor
  raptor_data_read32 : Raptor_lib/Data Storage/raptor_data_read  dataName='CMU2_CELL11_VOLT'  dataShape=Scalar  idxSource=Input  idxRow=1  idxCol=1
      settings: SourceProductName=Raptor
  raptor_data_read33 : Raptor_lib/Data Storage/raptor_data_read  dataName='CMU2_CELL12_VOLT'  dataShape=Scalar  idxSource=Input  idxRow=1  idxCol=1
      settings: SourceProductName=Raptor
  raptor_data_read34 : Raptor_lib/Data Storage/raptor_data_read  dataName='CMU2_CELL13_VOLT'  dataShape=Scalar  idxSource=Input  idxRow=1  idxCol=1
      settings: SourceProductName=Raptor
  raptor_data_read35 : Raptor_lib/Data Storage/raptor_data_read  dataName='CMU2_CELL14_VOLT'  dataShape=Scalar  idxSource=Input  idxRow=1  idxCol=1
      settings: SourceProductName=Raptor
  raptor_data_read36 : Raptor_lib/Data Storage/raptor_data_read  dataName='CMU2_CELL15_VOLT'  dataShape=Scalar  idxSource=Input  idxRow=1  idxCol=1
      settings: SourceProductName=Raptor
  raptor_data_read4 : Raptor_lib/Data Storage/raptor_data_read  dataName='CMU1_CELL05_VOLT'  dataShape=Scalar  idxSource=Input  idxRow=1  idxCol=1
      settings: SourceProductName=Raptor
  raptor_data_read42 : Raptor_lib/Data Storage/raptor_data_read  dataName='CMU2_CELL03_VOLT'  dataShape=Scalar  idxSource=Input  idxRow=1  idxCol=1
      settings: SourceProductName=Raptor
  raptor_data_read5 : Raptor_lib/Data Storage/raptor_data_read  dataName='CMU1_CELL06_VOLT'  dataShape=Scalar  idxSource=Input  idxRow=1  idxCol=1
      settings: SourceProductName=Raptor
  raptor_data_read53 : Raptor_lib/Data Storage/raptor_data_read  dataName='CMU2_CELL04_VOLT'  dataShape=Scalar  idxSource=Input  idxRow=1  idxCol=1
      settings: SourceProductName=Raptor
  raptor_data_read54 : Raptor_lib/Data Storage/raptor_data_read  dataName='CMU2_CELL05_VOLT'  dataShape=Scalar  idxSource=Input  idxRow=1  idxCol=1
      settings: SourceProductName=Raptor
  raptor_data_read55 : Raptor_lib/Data Storage/raptor_data_read  dataName='CMU2_CELL06_VOLT'  dataShape=Scalar  idxSource=Input  idxRow=1  idxCol=1
      settings: SourceProductName=Raptor
  raptor_data_read56 : Raptor_lib/Data Storage/raptor_data_read  dataName='CMU2_CELL07_VOLT'  dataShape=Scalar  idxSource=Input  idxRow=1  idxCol=1
      settings: SourceProductName=Raptor
  raptor_data_read57 : Raptor_lib/Data Storage/raptor_data_read  dataName='CMU2_CELL08_VOLT'  dataShape=Scalar  idxSource=Input  idxRow=1  idxCol=1
      settings: SourceProductName=Raptor
  raptor_data_read58 : Raptor_lib/Data Storage/raptor_data_read  dataName='CMU2_CELL09_VOLT'  dataShape=Scalar  idxSource=Input  idxRow=1  idxCol=1
      settings: SourceProductName=Raptor
  raptor_data_read59 : Raptor_lib/Data Storage/raptor_data_read  dataName='CMU2_CELL10_VOLT'  dataShape=Scalar  idxSource=Input  idxRow=1  idxCol=1
      settings: SourceProductName=Raptor
  raptor_data_read6 : Raptor_lib/Data Storage/raptor_data_read  dataName='CMU1_CELL07_VOLT'  dataShape=Scalar  idxSource=Input  idxRow=1  idxCol=1
      settings: SourceProductName=Raptor
  raptor_data_read7 : Raptor_lib/Data Storage/raptor_data_read  dataName='CMU1_CELL08_VOLT'  dataShape=Scalar  idxSource=Input  idxRow=1  idxCol=1
      settings: SourceProductName=Raptor
  raptor_data_read8 : Raptor_lib/Data Storage/raptor_data_read  dataName='CMU1_CELL09_VOLT'  dataShape=Scalar  idxSource=Input  idxRow=1  idxCol=1
      settings: SourceProductName=Raptor
  raptor_data_read9 : Raptor_lib/Data Storage/raptor_data_read  dataName='CMU1_CELL10_VOLT'  dataShape=Scalar  idxSource=Input  idxRow=1  idxCol=1
      settings: SourceProductName=Raptor
  Max : Outport
  Min : Outport  Port=2
  Max Order : Outport  Port=3
  Min Order : Outport  Port=4
  wires:
  Sort/2(Min) -> Min/1
  Mux/1 -> Sort/1(array)
  Sort/1(Max) -> Max/1
  raptor_data_read/1 -> Mux/1
  raptor_data_read1/1 -> Mux/2
  raptor_data_read2/1 -> Mux/3
  raptor_data_read3/1 -> Mux/4
  raptor_data_read4/1 -> Mux/5
  raptor_data_read5/1 -> Mux/6
  raptor_data_read6/1 -> Mux/7
  raptor_data_read7/1 -> Mux/8
  raptor_data_read8/1 -> Mux/9
  raptor_data_read9/1 -> Mux/10
  raptor_data_read10/1 -> Mux/11
  raptor_data_read11/1 -> Mux/12
  raptor_data_read12/1 -> Mux/13
  raptor_data_read13/1 -> Mux/14
  raptor_data_read14/1 -> Mux/15
  raptor_data_read30/1 -> Mux/16
  raptor_data_read31/1 -> Mux/17
  raptor_data_read42/1 -> Mux/18
  raptor_data_read53/1 -> Mux/19
  raptor_data_read54/1 -> Mux/20
  raptor_data_read55/1 -> Mux/21
  raptor_data_read56/1 -> Mux/22
  raptor_data_read57/1 -> Mux/23
  raptor_data_read58/1 -> Mux/24
  raptor_data_read59/1 -> Mux/25
  raptor_data_read32/1 -> Mux/26
  raptor_data_read33/1 -> Mux/27
  raptor_data_read34/1 -> Mux/28
  raptor_data_read35/1 -> Mux/29
  raptor_data_read36/1 -> Mux/30
  Sort/3(Max_order) -> Max Order/1
  Sort/4(Min_order) -> Min Order/1

== system EPT/Foreground_TimeBase_5ms/CAN/CAN3_exec/20CH_TCS/CH13_CH16_Rx/Convert_Byte2Data ==
  HighByte : Inport
  LowByte : Inport  Port=2
  Offset : Inport  Port=3
  Factor : Inport  Port=4
  Add2 : Sum
  Add5 : Sum
  Constant10 : Constant  Value=256
  Data Type Conversion10 : DataTypeConversion  OutDataTypeStr=double
  Divide6 : Product  Inputs=**
  Divide9 : Product  Inputs=**
  Data : Outport  VectorParamsAs1DForOutWhenUnconnected=off
  wires:
  Divide6/1 -> Add2/2
  LowByte/1 -> Add2/1
  Add5/1 -> Data Type Conversion10/1
  HighByte/1 -> Divide6/1
  Constant10/1 -> Divide6/2
  Divide9/1 -> Add5/1
  Add2/1 -> Divide9/1
  Data Type Conversion10/1 -> Data/1
  Factor/1 -> Divide9/2
  Offset/1 -> Add5/2

== system EPT/Foreground_TimeBase_5ms/CAN/CAN3_exec/20CH_TCS/CH13_CH16_Rx/Convert_Byte2Data1 ==
  HighByte : Inport
  LowByte : Inport  Port=2
  Offset : Inport  Port=3
  Factor : Inport  Port=4
  Add2 : Sum
  Add5 : Sum
  Constant10 : Constant  Value=256
  Data Type Conversion10 : DataTypeConversion  OutDataTypeStr=double
  Divide6 : Product  Inputs=**
  Divide9 : Product  Inputs=**
  Data : Outport  VectorParamsAs1DForOutWhenUnconnected=off
  wires:
  Offset/1 -> Add5/2
  Factor/1 -> Divide9/2
  Data Type Conversion10/1 -> Data/1
  Add2/1 -> Divide9/1
  Divide9/1 -> Add5/1
  Constant10/1 -> Divide6/2
  HighByte/1 -> Divide6/1
  Add5/1 -> Data Type Conversion10/1
  LowByte/1 -> Add2/1
  Divide6/1 -> Add2/2

== system EPT/Foreground_TimeBase_5ms/CAN/CAN3_exec/20CH_TCS/CH13_CH16_Rx/Convert_Byte2Data2 ==
  HighByte : Inport
  LowByte : Inport  Port=2
  Offset : Inport  Port=3
  Factor : Inport  Port=4
  Add2 : Sum
  Add5 : Sum
  Constant10 : Constant  Value=256
  Data Type Conversion10 : DataTypeConversion  OutDataTypeStr=double
  Divide6 : Product  Inputs=**
  Divide9 : Product  Inputs=**
  Data : Outport  VectorParamsAs1DForOutWhenUnconnected=off
  wires:
  Divide6/1 -> Add2/2
  LowByte/1 -> Add2/1
  Add5/1 -> Data Type Conversion10/1
  HighByte/1 -> Divide6/1
  Constant10/1 -> Divide6/2
  Divide9/1 -> Add5/1
  Add2/1 -> Divide9/1
  Data Type Conversion10/1 -> Data/1
  Factor/1 -> Divide9/2
  Offset/1 -> Add5/2

== system EPT/Foreground_TimeBase_5ms/CAN/CAN3_exec/20CH_TCS/CH13_CH16_Rx/Convert_Byte2Data3 ==
  HighByte : Inport
  LowByte : Inport  Port=2
  Offset : Inport  Port=3
  Factor : Inport  Port=4
  Add2 : Sum
  Add5 : Sum
  Constant10 : Constant  Value=256
  Data Type Conversion10 : DataTypeConversion  OutDataTypeStr=double
  Divide6 : Product  Inputs=**
  Divide9 : Product  Inputs=**
  Data : Outport  VectorParamsAs1DForOutWhenUnconnected=off
  wires:
  Offset/1 -> Add5/2
  Factor/1 -> Divide9/2
  Data Type Conversion10/1 -> Data/1
  Add2/1 -> Divide9/1
  Divide9/1 -> Add5/1
  Constant10/1 -> Divide6/2
  HighByte/1 -> Divide6/1
  Add5/1 -> Data Type Conversion10/1
  LowByte/1 -> Add2/1
  Divide6/1 -> Add2/2

== system EPT/Foreground_TimeBase_5ms/CAN/CAN3_exec/20CH_TCS/CH17_CH20_Rx1/Convert_Byte2Data ==
  HighByte : Inport
  LowByte : Inport  Port=2
  Offset : Inport  Port=3
  Factor : Inport  Port=4
  Add2 : Sum
  Add5 : Sum
  Constant10 : Constant  Value=256
  Data Type Conversion10 : DataTypeConversion  OutDataTypeStr=double
  Divide6 : Product  Inputs=**
  Divide9 : Product  Inputs=**
  Data : Outport  VectorParamsAs1DForOutWhenUnconnected=off
  wires:
  Divide6/1 -> Add2/2
  LowByte/1 -> Add2/1
  Add5/1 -> Data Type Conversion10/1
  HighByte/1 -> Divide6/1
  Constant10/1 -> Divide6/2
  Divide9/1 -> Add5/1
  Add2/1 -> Divide9/1
  Data Type Conversion10/1 -> Data/1
  Factor/1 -> Divide9/2
  Offset/1 -> Add5/2

== system EPT/Foreground_TimeBase_5ms/CAN/CAN3_exec/20CH_TCS/CH17_CH20_Rx1/Convert_Byte2Data1 ==
  HighByte : Inport
  LowByte : Inport  Port=2
  Offset : Inport  Port=3
  Factor : Inport  Port=4
  Add2 : Sum
  Add5 : Sum
  Constant10 : Constant  Value=256
  Data Type Conversion10 : DataTypeConversion  OutDataTypeStr=double
  Divide6 : Product  Inputs=**
  Divide9 : Product  Inputs=**
  Data : Outport  VectorParamsAs1DForOutWhenUnconnected=off
  wires:
  Offset/1 -> Add5/2
  Factor/1 -> Divide9/2
  Data Type Conversion10/1 -> Data/1
  Add2/1 -> Divide9/1
  Divide9/1 -> Add5/1
  Constant10/1 -> Divide6/2
  HighByte/1 -> Divide6/1
  Add5/1 -> Data Type Conversion10/1
  LowByte/1 -> Add2/1
  Divide6/1 -> Add2/2

== system EPT/Foreground_TimeBase_5ms/CAN/CAN3_exec/20CH_TCS/CH17_CH20_Rx1/Convert_Byte2Data2 ==
  HighByte : Inport
  LowByte : Inport  Port=2
  Offset : Inport  Port=3
  Factor : Inport  Port=4
  Add2 : Sum
  Add5 : Sum
  Constant10 : Constant  Value=256
  Data Type Conversion10 : DataTypeConversion  OutDataTypeStr=double
  Divide6 : Product  Inputs=**
  Divide9 : Product  Inputs=**
  Data : Outport  VectorParamsAs1DForOutWhenUnconnected=off
  wires:
  Divide6/1 -> Add2/2
  LowByte/1 -> Add2/1
  Add5/1 -> Data Type Conversion10/1
  HighByte/1 -> Divide6/1
  Constant10/1 -> Divide6/2
  Divide9/1 -> Add5/1
  Add2/1 -> Divide9/1
  Data Type Conversion10/1 -> Data/1
  Factor/1 -> Divide9/2
  Offset/1 -> Add5/2

== system EPT/Foreground_TimeBase_5ms/CAN/CAN3_exec/20CH_TCS/CH17_CH20_Rx1/Convert_Byte2Data3 ==
  HighByte : Inport
  LowByte : Inport  Port=2
  Offset : Inport  Port=3
  Factor : Inport  Port=4
  Add2 : Sum
  Add5 : Sum
  Constant10 : Constant  Value=256
  Data Type Conversion10 : DataTypeConversion  OutDataTypeStr=double
  Divide6 : Product  Inputs=**
  Divide9 : Product  Inputs=**
  Data : Outport  VectorParamsAs1DForOutWhenUnconnected=off
  wires:
  Offset/1 -> Add5/2
  Factor/1 -> Divide9/2
  Data Type Conversion10/1 -> Data/1
  Add2/1 -> Divide9/1
  Divide9/1 -> Add5/1
  Constant10/1 -> Divide6/2
  HighByte/1 -> Divide6/1
  Add5/1 -> Data Type Conversion10/1
  LowByte/1 -> Add2/1
  Divide6/1 -> Add2/2

== system EPT/Foreground_TimeBase_5ms/CAN/CAN3_exec/20CH_TCS/CH1_CH4_Rx/Convert_Byte2Data ==
  HighByte : Inport
  LowByte : Inport  Port=2
  Offset : Inport  Port=3
  Factor : Inport  Port=4
  Add2 : Sum
  Add5 : Sum
  Constant10 : Constant  Value=256
  Data Type Conversion10 : DataTypeConversion  OutDataTypeStr=double
  Divide6 : Product  Inputs=**
  Divide9 : Product  Inputs=**
  Data : Outport  VectorParamsAs1DForOutWhenUnconnected=off
  wires:
  Divide6/1 -> Add2/2
  LowByte/1 -> Add2/1
  Add5/1 -> Data Type Conversion10/1
  HighByte/1 -> Divide6/1
  Constant10/1 -> Divide6/2
  Divide9/1 -> Add5/1
  Add2/1 -> Divide9/1
  Data Type Conversion10/1 -> Data/1
  Factor/1 -> Divide9/2
  Offset/1 -> Add5/2

== system EPT/Foreground_TimeBase_5ms/CAN/CAN3_exec/20CH_TCS/CH1_CH4_Rx/Convert_Byte2Data1 ==
  HighByte : Inport
  LowByte : Inport  Port=2
  Offset : Inport  Port=3
  Factor : Inport  Port=4
  Add2 : Sum
  Add5 : Sum
  Constant10 : Constant  Value=256
  Data Type Conversion10 : DataTypeConversion  OutDataTypeStr=double
  Divide6 : Product  Inputs=**
  Divide9 : Product  Inputs=**
  Data : Outport  VectorParamsAs1DForOutWhenUnconnected=off
  wires:
  Offset/1 -> Add5/2
  Factor/1 -> Divide9/2
  Data Type Conversion10/1 -> Data/1
  Add2/1 -> Divide9/1
  Divide9/1 -> Add5/1
  Constant10/1 -> Divide6/2
  HighByte/1 -> Divide6/1
  Add5/1 -> Data Type Conversion10/1
  LowByte/1 -> Add2/1
  Divide6/1 -> Add2/2
